simulink model "shell_eco_mainV9_track"  (R2023b)
settings: Solver=ode23tb  StartTime=0.0  StopTime=t_end  MaxStep=0.1  RelTol=1e-3
undefined symbols (not defined in the file): A, Cd, Crr, effic_drive, effic_engine, EngineRPM_map, EngineTorque_map, g, G, lap_distance, LHV, m, r_w, rho, RPM_idle, RPM_max, total_dist, track_grade, track_v_limit, track_x_breaks, track_zone, v0, v_high_on, v_low_on, v_target, x0
settings Model: Creator=canfi  LastModifiedBy=canfi
settings SolverCC: MaxConsecutiveZCs=10000  ZeroCrossAlgorithm=Adaptive
settings DebuggingCC: IgnoredZcDiagnostic=none

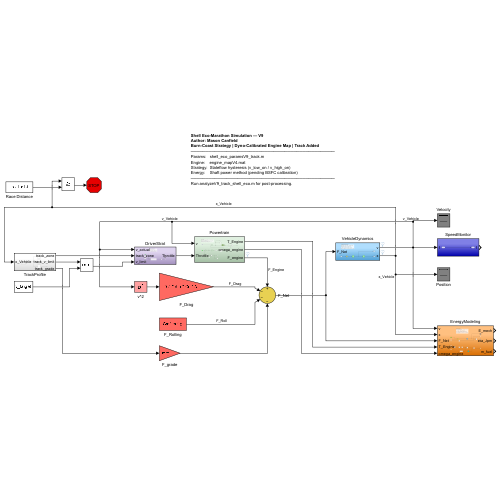
[thumbnail: Simulink's stored preview of the top-level diagram]
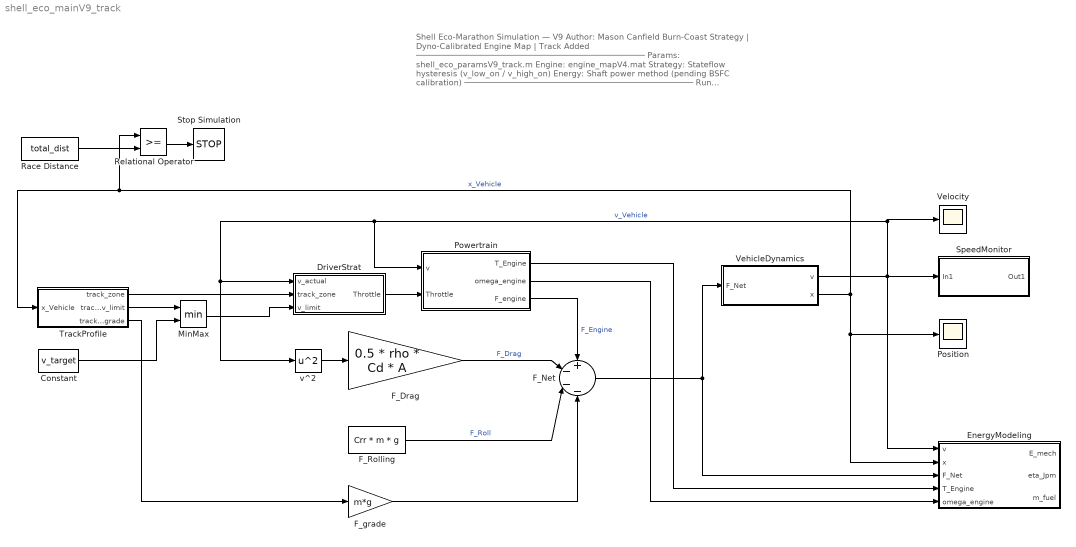
== system shell_eco_mainV9_track ==
  note: Shell Eco-Marathon Simulation — V9
      | Author: Mason Canfield
      | Burn-Coast Strategy | Dyno-Calibrated Engine Map | Track Added
      | ─────────────────────────────────────────────────
      | Params: shell_eco_paramsV9_track.m
      | Engine: engine_mapV4.mat
      | Strategy: Stateflow hysteresis (v_low_on / v_high_on)
      | Energy: Shaft power method (pending BSFC calibration)
      | ─────────────────────────────────────────────────
      | Run analyzeV9_track_shell_eco.m for post-processing.
  Constant : Constant  Value=v_target
  DriverStrat : Subsystem
  EnergyModeling : Subsystem
  F_Drag : Gain  Gain=0.5 * rho * Cd * A
  F_Net : Sum  Inputs=+---
  F_Rolling : Constant  Value=Crr * m * g
  F_grade : Gain  Gain=m*g
  MinMax : MinMax  Inputs=2
  Position : Scope
  Powertrain : Subsystem
  Race Distance : Constant  Value=total_dist
  Relational Operator : RelationalOperator  OutDataTypeStr=boolean  RndMeth=Simplest  InputSameDT=off
  SpeedMonitor : Subsystem
  Stop Simulation : Stop
  TrackProfile : Subsystem
  VehicleDynamics : Subsystem
  Velocity : Scope
  v^2 : Math  Operator=square
  wires:
  DriverStrat/1(Throttle) -> Powertrain/2(Throttle)
  VehicleDynamics/2(x) -> TrackProfile/1(x_Vehicle), Relational Operator/1, Position/1, EnergyModeling/2(x)  "x_Vehicle"
  VehicleDynamics/1(v) -> Velocity/1, Powertrain/1(v), v^2/1, DriverStrat/1(v_actual), SpeedMonitor/1(In1), EnergyModeling/1(v)  "v_Vehicle"
  Powertrain/3(F_engine) -> F_Net/1  "F_Engine"
  v^2/1 -> F_Drag/1
  F_Net/1 -> EnergyModeling/3(F_Net), VehicleDynamics/1(F_Net)
  F_Rolling/1 -> F_Net/3  "F_Roll"
  F_Drag/1 -> F_Net/2  "F_Drag"
  Powertrain/1(T_Engine) -> EnergyModeling/4(T_Engine)
  Powertrain/2(omega_engine) -> EnergyModeling/5(omega_engine)
  TrackProfile/3(track_grade) -> F_grade/1
  F_grade/1 -> F_Net/4
  Race Distance/1 -> Relational Operator/2
  Relational Operator/1 -> Stop Simulation/1
  TrackProfile/2(track_v_limit) -> MinMax/1
  Constant/1 -> MinMax/2
  MinMax/1 -> DriverStrat/3(v_limit)
  TrackProfile/1(track_zone) -> DriverStrat/2(track_zone)

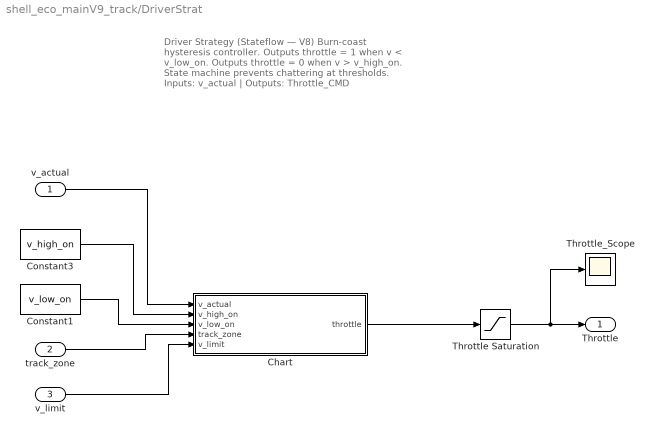
== system shell_eco_mainV9_track/DriverStrat ==
  note: Driver Strategy (Stateflow — V8)
      | Burn-coast hysteresis controller.
      | Outputs throttle = 1 when v < v_low_on.
      | Outputs throttle = 0 when v > v_high_on.
      | State machine prevents chattering at thresholds.
      | Inputs: v_actual | Outputs: Throttle_CMD
  v_actual : Inport
  track_zone : Inport  Port=2
  v_limit : Inport  Port=3
  Chart : Stateflow chart  TreatAsAtomicUnit=on  SystemSampleTime=0.1
      settings: PortSchema="{\"entries\":[{\"content\":{\"sides\":[{\"content\":{\"connectorIds\":[\"In1\",\"In2\",\"In3\",\"In5\",\"In4\"]},\"type\":\"ConnectorPlacement.EquallySpacedRectSide\",\"uuid\":\"95d78ea3-a0eb-4612-ac09-2b338d40569c\"},{\"content\":{\"connectorIds\":[\"Out1\"],\"side\":\"RIGHT\"},\"type\":\"ConnectorPlacement.EquallySpacedRectSide\",\"uuid\":\"8de828c1-ab5e-43e5-b354-384a79ff888e\"},{\"content\":{\"side\":\"TOP\"},\"type\":\"ConnectorPlacement.EquallySpacedRectSide\",\"uuid\":\"c3a3f22b-c6ed-42e6-a0a1-b1648d0d87a6\"}]},\"type\":\"ConnectorPlacement.EquallySpacedConnector\",\"uuid\":\"57e09216-1d25-414b-ae5f-ef7ae26cf522\"}],\"packageUris\":[\"http://schema.mathworks.com/mf0/Connector/R2020b\"],\"version\":\"1.0\"}"
  Constant1 : Constant  Value=v_low_on
  Constant3 : Constant  Value=v_high_on
  Throttle Saturation : Saturate  UpperLimit=1  LowerLimit=0
  Throttle_Scope : Scope
  Throttle : Outport
  wires:
  v_actual/1 -> Chart/1(v_actual)
  Constant1/1 -> Chart/3(v_low_on)
  Constant3/1 -> Chart/2(v_high_on)
  Chart/1(throttle) -> Throttle Saturation/1
  Throttle Saturation/1 -> Throttle_Scope/1, Throttle/1
  track_zone/1 -> Chart/5(track_zone)
  v_limit/1 -> Chart/4(v_limit)

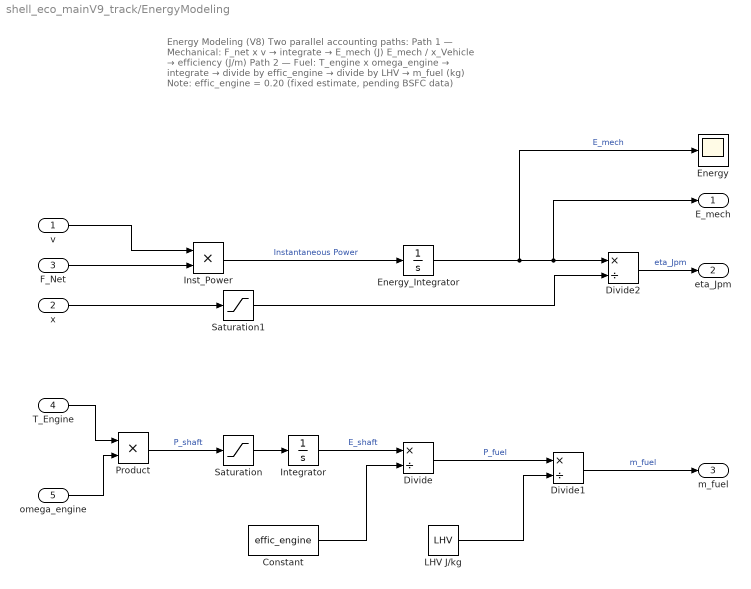
== system shell_eco_mainV9_track/EnergyModeling ==
  note: Energy Modeling (V8)
      | Two parallel accounting paths:
      | Path 1 — Mechanical: F_net x v → integrate → E_mech (J)
      | E_mech / x_Vehicle → efficiency (J/m)
      | Path 2 — Fuel: T_engine x omega_engine → integrate
      | → divide by effic_engine → divide by LHV
      | → m_fuel (kg)
      | Note: effic_engine = 0.20 (fixed estimate, pending BSFC data)
  v : Inport
  x : Inport  Port=2
  F_Net : Inport  Port=3
  T_Engine : Inport  Port=4
  omega_engine : Inport  Port=5
  Constant : Constant  Value=effic_engine
  Divide : Product  Inputs=*/
  Divide1 : Product  Inputs=*/
  Divide2 : Product  Inputs=*/
  Energy : Scope
  Energy_Integrator : Integrator
  Inst_Power : Product
  Integrator : Integrator
  LHV J/kg : Constant  Value=LHV
  Product : Product
  Saturation : Saturate  UpperLimit=inf  LowerLimit=0
  Saturation1 : Saturate  UpperLimit=inf  LowerLimit=0.001
  E_mech : Outport
  eta_Jpm : Outport  Port=2
  m_fuel : Outport  Port=3
  wires:
  v/1 -> Inst_Power/1
  F_Net/1 -> Inst_Power/2
  Inst_Power/1 -> Energy_Integrator/1  "Instantaneous Power"
  Energy_Integrator/1 -> E_mech/1, Divide2/1, Energy/1  "E_mech"
  LHV J/kg/1 -> Divide1/2
  Divide1/1 -> m_fuel/1  "m_fuel"
  T_Engine/1 -> Product/1
  omega_engine/1 -> Product/2
  Product/1 -> Saturation/1  "P_shaft"
  Constant/1 -> Divide/2
  Divide/1 -> Divide1/1  "P_fuel"
  Integrator/1 -> Divide/1  "E_shaft"
  Divide2/1 -> eta_Jpm/1  "eta_Jpm"
  Saturation/1 -> Integrator/1
  x/1 -> Saturation1/1
  Saturation1/1 -> Divide2/2

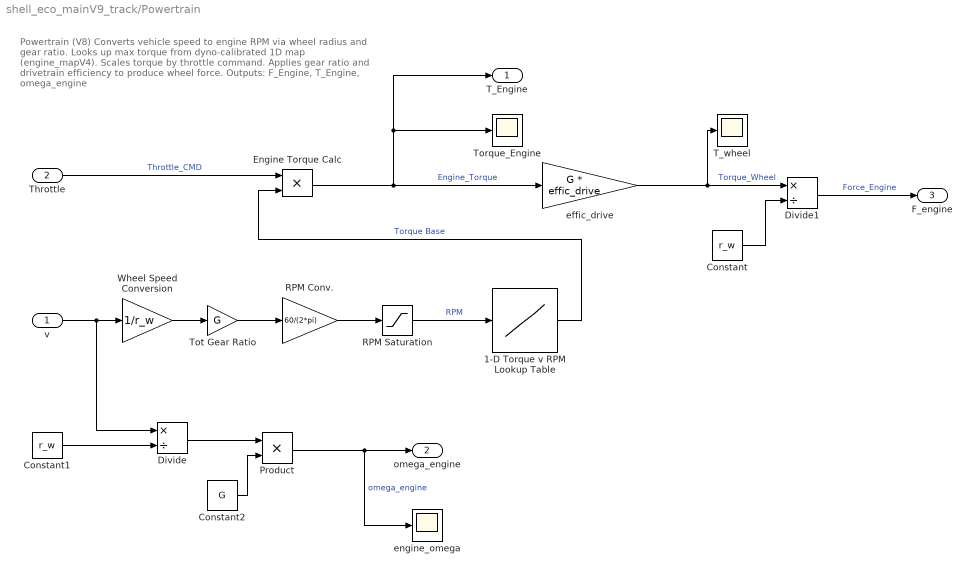
== system shell_eco_mainV9_track/Powertrain ==
  note: Powertrain (V8)
      | Converts vehicle speed to engine RPM via wheel radius and gear ratio.
      | Looks up max torque from dyno-calibrated 1D map (engine_mapV4).
      | Scales torque by throttle command.
      | Applies gear ratio and drivetrain efficiency to produce wheel force.
      | Outputs: F_Engine, T_Engine, omega_engine
  v : Inport
  Throttle : Inport  Port=2
  1-D Torque v RPM Lookup Table : Lookup_n-D  NumberOfTableDimensions=1  BreakpointsForDimension1=EngineRPM_map  Table=EngineTorque_map  ExtrapMethod=Clip  InternalRulePriority=Speed  RndMeth=Simplest
  Constant : Constant  Value=r_w
  Constant1 : Constant  Value=r_w
  Constant2 : Constant  Value=G
  Divide : Product  Inputs=*/
  Divide1 : Product  Inputs=*/
  Engine Torque Calc : Product
  Product : Product
  RPM Conv. : Gain  Gain=60/(2*pi)
  RPM Saturation : Saturate  UpperLimit=RPM_max  LowerLimit=RPM_idle
  T_wheel : Scope
  Torque_Engine : Scope
  Tot Gear Ratio : Gain  Gain=G
  Wheel Speed Conversion : Gain  Gain=1/r_w
  effic_drive : Gain  Gain=G * effic_drive
  engine_omega : Scope
  T_Engine : Outport
  omega_engine : Outport  Port=2
  F_engine : Outport  Port=3
  wires:
  Wheel Speed Conversion/1 -> Tot Gear Ratio/1
  Tot Gear Ratio/1 -> RPM Conv./1
  v/1 -> Divide/1, Wheel Speed Conversion/1
  RPM Conv./1 -> RPM Saturation/1
  1-D Torque v RPM Lookup Table/1 -> Engine Torque Calc/2  "Torque Base"
  Throttle/1 -> Engine Torque Calc/1  "Throttle_CMD"
  Engine Torque Calc/1 -> T_Engine/1, Torque_Engine/1, effic_drive/1  "Engine_Torque"
  Divide1/1 -> F_engine/1  "Force_Engine"
  RPM Saturation/1 -> 1-D Torque v RPM Lookup Table/1  "RPM"
  effic_drive/1 -> T_wheel/1, Divide1/1  "Torque_Wheel"
  Constant/1 -> Divide1/2
  Constant1/1 -> Divide/2
  Divide/1 -> Product/1
  Constant2/1 -> Product/2
  Product/1 -> engine_omega/1, omega_engine/1  "omega_engine"

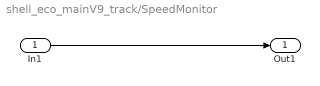
== system shell_eco_mainV9_track/SpeedMonitor ==
  In1 : Inport
  Out1 : Outport
  wires:
  In1/1 -> Out1/1

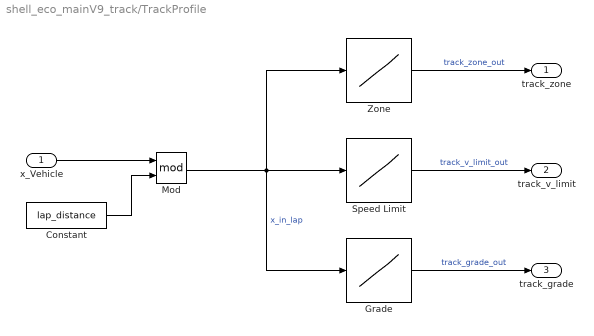
== system shell_eco_mainV9_track/TrackProfile ==
  x_Vehicle : Inport
  Constant : Constant  Value=lap_distance
  Grade : Lookup_n-D  NumberOfTableDimensions=1  BreakpointsForDimension1=track_x_breaks  Table=track_grade  InterpMethod=Flat  InternalRulePriority=Speed  RndMeth=Simplest
  Mod : Math  Operator=mod
  Speed Limit : Lookup_n-D  NumberOfTableDimensions=1  BreakpointsForDimension1=track_x_breaks  Table=track_v_limit  InterpMethod=Flat  InternalRulePriority=Speed  RndMeth=Simplest
  Zone : Lookup_n-D  NumberOfTableDimensions=1  BreakpointsForDimension1=track_x_breaks  Table=track_zone  InterpMethod=Flat  InternalRulePriority=Speed  RndMeth=Simplest
  track_zone : Outport
  track_v_limit : Outport  Port=2
  track_grade : Outport  Port=3
  wires:
  x_Vehicle/1 -> Mod/1
  Constant/1 -> Mod/2
  Mod/1 -> Speed Limit/1, Zone/1, Grade/1  "x_in_lap"
  Zone/1 -> track_zone/1  "track_zone_out"
  Speed Limit/1 -> track_v_limit/1  "track_v_limit_out"
  Grade/1 -> track_grade/1  "track_grade_out"

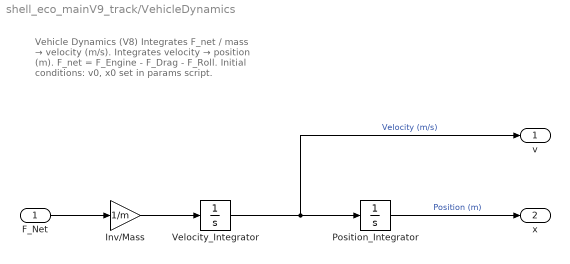
== system shell_eco_mainV9_track/VehicleDynamics ==
  note: Vehicle Dynamics (V8)
      | Integrates F_net / mass → velocity (m/s).
      | Integrates velocity → position (m).
      | F_net = F_Engine - F_Drag - F_Roll.
      | Initial conditions: v0, x0 set in params script.
  F_Net : Inport
  Inv/Mass : Gain  Gain=1/m
  Position_Integrator : Integrator  InitialCondition=x0
  Velocity_Integrator : Integrator  InitialCondition=v0
  v : Outport
  x : Outport  Port=2
  wires:
  Inv/Mass/1 -> Velocity_Integrator/1
  Velocity_Integrator/1 -> v/1, Position_Integrator/1  "Velocity (m/s)"
  Position_Integrator/1 -> x/1  "Position (m)"
  F_Net/1 -> Inv/Mass/1

== stateflow chart shell_eco_mainV9_track/DriverStrat/Chart ==
  settings: updateMethod=DISCRETE  sampleTime=0.1
  state BURN
    entry: throttle = 1;
  state COAST
    entry: throttle = 0;
  state CRUISE
    during:
    if v_actual < v_limit - 0.1
    throttle = 1;
    elseif v_actual > v_limit + 0.1
    throttle = 0;
    end
  (default) -> BURN
  BURN -> COAST [order 1] : [track_zone == 1 && v_actual >= v_high_on]
  COAST -> BURN [order 1] : [track_zone == 1 && v_actual <= v_low_on]
  CRUISE -> BURN [order 1] : [[track_zone == 1 && v_actual <= v_low_on]]
  BURN -> CRUISE [order 2] : [[track_zone ~= 1]]
  COAST -> CRUISE [order 2] : [[track_zone ~= 1]]
  CRUISE -> COAST [order 2] : [[track_zone == 1 && v_actual >= v_high_on]]
  data: v_actual input; v_high_on input; v_low_on input; throttle output; v_limit input double; track_zone input double
